simulink model "Lab1_6B"  (R2018a)
settings: Solver=VariableStepAuto  StartTime=0.0  StopTime=180  RelTol=1e-3
settings Model: Creator=melab2  LastModifiedBy=rahul

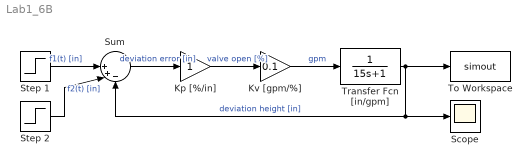
== system Lab1_6B ==
  Kp [%/in] : Gain
  Kv [gpm/%] : Gain  Gain=0.1
  Scope : Scope
  "Step 1 " : Step  SampleTime=0
  Step 2 : Step  Time=75  After=-2  SampleTime=0
  Sum : Sum  Inputs=||++-
  To Workspace : ToWorkspace  VariableName=simout  SampleTime=-1
  Transfer Fcn [in/gpm] : TransferFcn  Denominator=[15 1]
  wires:
  Sum/1 -> Kp [%/in]/1  "deviation error [in]"
  Kp [%/in]/1 -> Kv [gpm/%]/1  "valve open [%]"
  Kv [gpm/%]/1 -> Transfer Fcn [in/gpm]/1  "gpm"
  Transfer Fcn [in/gpm]/1 -> Sum/3, Scope/1, To Workspace/1  "deviation height [in]"
  "Step 1 "/1 -> Sum/1  "f1(t) [in]"
  Step 2/1 -> Sum/2  "f2(t) [in]"
